simulink model "siso_pitch_break"  (R2026a)
settings: Solver=VariableStepAuto  StopTime=10
undefined symbols (not defined in the file or in its folder): P
libraries: slpidlib x2, dspfdesign x1, simulink x1
settings Model: Creator=devinbellll  LastModifiedBy=devinbellll

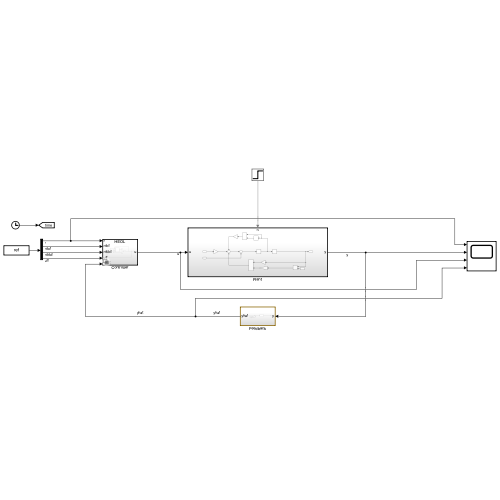
[thumbnail: Simulink's stored preview of the top-level diagram]
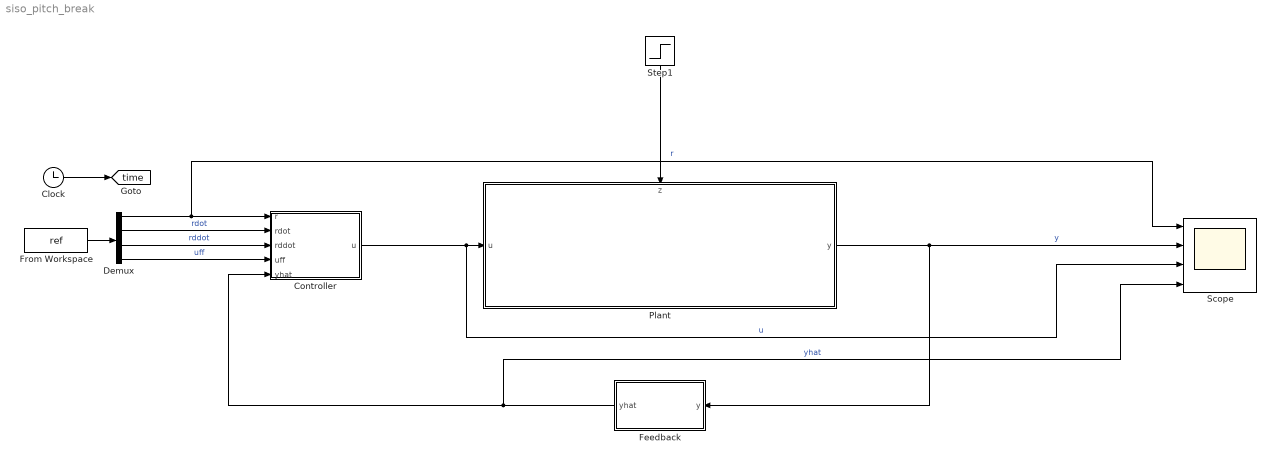
== system siso_pitch_break ==
  Clock : Clock
  Controller : Subsystem  Variant=on  VariantControlMode=label  LabelModeActiveChoice=HEOL
  Demux : Demux
  Feedback : Subsystem
  From Workspace : FromWorkspace  VariableName=ref
  Plant : Subsystem
      settings: PortSchema="{\"entries\":[{\"content\":{\"sides\":[{\"content\":{\"connectorIds\":[\"In1\"]},\"type\":\"ConnectorPlacement.EquallySpacedRectSide\",\"uuid\":\"c97da850-f89b-4091-b1f5-05dae9f68cd3\"},{\"content\":{\"connectorIds\":[\"Out1\"],\"side\":\"RIGHT\"},\"type\":\"ConnectorPlacement.EquallySpacedRectSide\",\"uuid\":\"c303f837-7d2b-4813-8ee2-fdf25e492c4f\"},{\"content\":{\"connectorIds\":[\"In2\"],\"side\":\"TOP\"},\"type\":\"ConnectorPlacement.EquallySpacedRectSide\",\"uuid\":\"7bfe1516-e3c7-473c-aa51-3e09351ce59e\"}]},\"type\":\"ConnectorPlacement.EquallySpacedConnector\",\"uuid\":\"d0f3ac38-9d06-47ac-81ff-254dc0ebc63c\"}],\"packageUris\":[\"http://schema.mathworks.com/mf0/Connector/R2020b\"],\"version\":\"1.0\"}"
  Scope : Scope  NumInputPorts=4
      settings: ActiveDisplayYMinimum=-0.1850564356772344  ActiveDisplayYMaximum=0.35875841753576132
  Step1 : Step  Time=5  FinalValue=10  SampleTime=0
  tag scope: time=global
  wires:
  Plant/1(y) -> Feedback/1(y), Scope/2  "y"
  Clock/1 -> [time]
  Demux/1 -> Controller/1(r), Scope/1  "r"
  Step1/1 -> Plant/2(z)
  Feedback/1(yhat) -> Controller/5(yhat), Scope/4  "yhat"
  From Workspace/1 -> Demux/1
  Demux/2 -> Controller/2(rdot)  "rdot"
  Demux/3 -> Controller/3(rddot)  "rddot"
  Demux/4 -> Controller/4(uff)  "uff"
  Controller/1(u) -> Plant/1(u), Scope/3  "u"

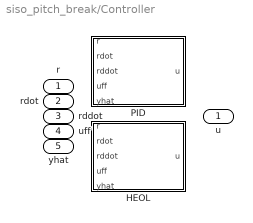
== system siso_pitch_break/Controller ==
  r : Inport
  rdot : Inport  Port=2
  rddot : Inport  Port=3
  uff : Inport  Port=4
  yhat : Inport  Port=5
  HEOL : Subsystem  VariantControl=HEOL
  PID : Subsystem  VariantControl=PID
  u : Outport

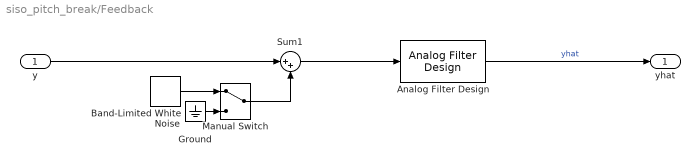
== system siso_pitch_break/Feedback ==
  y : Inport
  Analog Filter Design : dspfdesign/Analog Filter Design  method=Butterworth  filttype=Lowpass  N=2  Wlo=P.wf  Whi=80  Rp=2  Rs=40
  Band-Limited White Noise : simulink/Sources/Band-Limited White Noise  Cov=P.noise_pw  Ts=P.Ts  seed=P.seed
  Ground : Ground
  Manual Switch : ManualSwitch
  Sum1 : Sum  Inputs=|++
  yhat : Outport
  wires:
  y/1 -> Sum1/1
  Manual Switch/1 -> Sum1/2
  Band-Limited White Noise/1 -> Manual Switch/1
  Ground/1 -> Manual Switch/2
  Analog Filter Design/1 -> yhat/1  "yhat"
  Sum1/1 -> Analog Filter Design/1

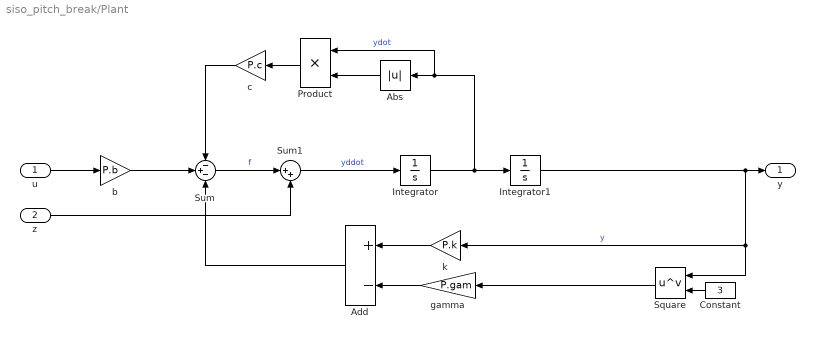
== system siso_pitch_break/Plant ==
  u : Inport
  z : Inport  Port=2
  Abs : Abs  SaturateOnIntegerOverflow=off
  Add : Sum  Inputs=+-
  Constant : Constant  Value=3
  Integrator : Integrator
  Integrator1 : Integrator
  Product : Product
  Square : Math  Operator=pow
  Sum : Sum  Inputs=-+-
  Sum1 : Sum  Inputs=|++
  b : Gain  Gain=P.b
  c : Gain  Gain=P.c
  gamma : Gain  Gain=P.gam
  k : Gain  Gain=P.k
  y : Outport
  wires:
  u/1 -> b/1
  b/1 -> Sum/2
  Abs/1 -> Product/2
  Sum/1 -> Sum1/1  "f"
  Integrator/1 -> Product/1, Abs/1, Integrator1/1  "ydot"
  Integrator1/1 -> Square/1, k/1, y/1  "y"
  Product/1 -> c/1
  c/1 -> Sum/1
  Add/1 -> Sum/3
  gamma/1 -> Add/2
  Square/1 -> gamma/1
  Constant/1 -> Square/2
  k/1 -> Add/1
  Sum1/1 -> Integrator/1  "yddot"
  z/1 -> Sum1/2

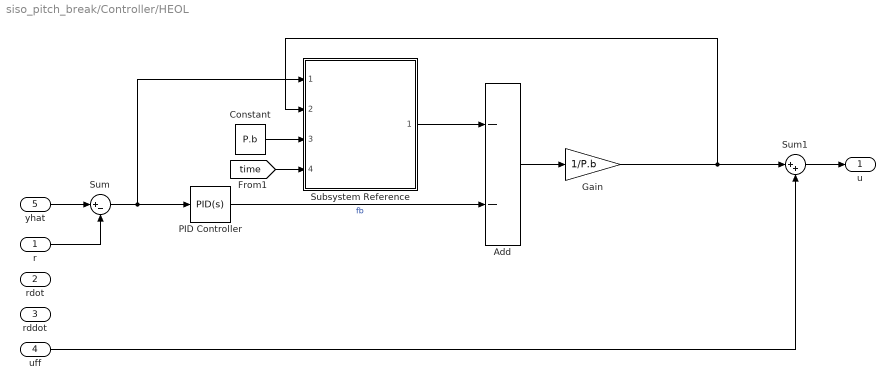
== system siso_pitch_break/Controller/HEOL ==
  r : Inport
  rdot : Inport  Port=2
  rddot : Inport  Port=3
  uff : Inport  Port=4
  yhat : Inport  Port=5
  Add : Sum  Inputs=--
  Constant : Constant  Value=P.b
  Gain : Gain  Gain=1/P.b
  PID Controller : slpidlib/PID Controller  Controller=PID  Form=Parallel  TimeDomain=Continuous-time  UseExternalTs=off  SampleTime=-1  IntegratorMethod=Forward Euler  FilterMethod=Forward Euler  ControllerParametersSource=internal  P=P.Kp  I=P.Ki  UseKiTs=off  D=P.Kd  UseExternalDerivativeSource=off  N=P.N  UseFilter=on  TunerSelectOption=Transfer Function Based (PID Tuner App)  InitialConditionSource=internal  InitialConditionForIntegrator=0  InitialConditionForFilter=0  DifferentiatorICPrevScaledInput=0  ExternalReset=none  TrackingMode=off  Kt=1  LimitOutput=off  SatLimitsSource=internal  UpperSaturationLimit=inf  LowerSaturationLimit=-inf  LinearizeAsGain=on  AntiWindupMode=none  Kb=1  LimitIntegrator=off  UpperIntegratorSaturationLimit=inf  LowerIntegratorSaturationLimit=-inf  POutMin=[]  POutMax=[]  IOutMin=[]  IOutMax=[]  DOutMin=[]  DOutMax=[]  NOutMin=[]  NOutMax=[]  SumOutMin=[]  SumOutMax=[]  SaturationOutMin=[]  SaturationOutMax=[]  PParamMin=[]  PParamMax=[]  IParamMin=[]  IParamMax=[]  DParamMin=[]  DParamMax=[]  NParamMin=[]  NParamMax=[]  KbParamMin=[]  KbParamMax=[]  KtParamMin=[]  KtParamMax=[]  KbOutMin=[]  KbOutMax=[]  KtOutMin=[]  KtOutMax=[]  IntegratorOutMin=[]  IntegratorOutMax=[]  FilterOutMin=[]  FilterOutMax=[]  SumI1OutMin=[]  SumI1OutMax=[]  SumI2OutMin=[]  SumI2OutMax=[]  SumI3OutMin=[]  SumI3OutMax=[]  SumI4OutMin=[]  SumI4OutMax=[]  SumDOutMin=[]  SumDOutMax=[]  DifferentiatorOutMin=[]  DifferentiatorOutMax=[]  FilterDiffOutCoefMin=[]  FilterDiffOutCoefMax=[]  ReciprocalOutMin=[]  ReciprocalOutMax=[]  SumDenOutMin=[]  SumDenOutMax=[]  SumNumOutMin=[]  SumNumOutMax=[]  DivideOutMin=[]  DivideOutMax=[]  UdiffTsProdOutMin=[]  UdiffTsProdOutMax=[]  NTsProdOutMin=[]  NTsProdOutMax=[]  UintegralTsProdOutMin=[]  UintegralTsProdOutMax=[]  UngainTsProdOutMin=[]  UngainTsProdOutMax=[]  ClampingZeroOutDataTypeStr=Inherit: Inherit via back propagation  ClampingZeroOutMin=[]  ClampingZeroOutMax=[]  FilterDenConstantOutDataTypeStr=Inherit: Inherit via back propagation  FilterDenConstantOutMin=[]  FilterDenConstantOutMax=[]  PCopyOutDataTypeStr=Inherit: Inherit via back propagation  PCopyOutMin=[]  PCopyOutMax=[]  NCopyOutDataTypeStr=Inherit: Inherit via back propagation  NCopyOutMin=[]  NCopyOutMax=[]  IntegratorContinuousStateAttributes=''  IntegratorStateMustResolveToSignalObject=off  IntegratorRTWStateStorageClass=Auto  FilterContinuousStateAttributes=''  FilterStateMustResolveToSignalObject=off  FilterRTWStateStorageClass=Auto  ParallelPVariant=InternalParameters  IdealPVariant=Disabled  IVariant=InternalParameters  DVariant=InternalParameters  IntegratorVariant=Continuous  SatVariant=Disabled  AWVariant=Passthrough  PCopyVariant=Disabled  TRVariant=Disabled  FdbkBlocksVariant=Forward  IdealPFdbkVariant=Disabled  SatFdbkVariant=Disabled  DerivativeFilterVariant=ContFilter  NVariant=InternalParameters  NCopyVariant=Disabled  FilterICVariant=InternalICsFilter  IntegratorICVariant=InternalICs  ExternalResetVariant=Disabled  TRSumVariant=Passthrough  SumFdbkVariant=Disabled  SumVariant=Sum_PID  TsampFilterVariant=InternalTs  TsampNgainVariant=Passthrough  TsampIntegralVariant=Disabled_SignalSpec  ExternalSaturationOutDataTypeStr=Inherit: Same as second input  DerivativeSourceVariant=ErrorSignal  PreIntVariant=InternalPreInt
  Subsystem Reference : Subsystem  ReferencedSubsystem=mfc_F_est_cont
  Sum : Sum  Inputs=|+-
  Sum1 : Sum  Inputs=|++
  u : Outport
  wires:
  uff/1 -> Sum1/2
  Sum1/1 -> u/1
  PID Controller/1 -> Add/2  "fb"
  r/1 -> Sum/2
  Sum/1 -> Subsystem Reference/1, PID Controller/1
  [time] -> Subsystem Reference/4
  yhat/1 -> Sum/1
  Constant/1 -> Subsystem Reference/3
  Gain/1 -> Subsystem Reference/2, Sum1/1
  Subsystem Reference/1 -> Add/1
  Add/1 -> Gain/1

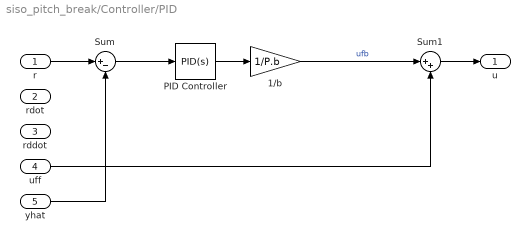
== system siso_pitch_break/Controller/PID ==
  r : Inport
  rdot : Inport  Port=2
  rddot : Inport  Port=3
  uff : Inport  Port=4
  yhat : Inport  Port=5
  1/b : Gain  Gain=1/P.b
  PID Controller : slpidlib/PID Controller  Controller=PID  Form=Parallel  TimeDomain=Continuous-time  UseExternalTs=off  SampleTime=-1  IntegratorMethod=Forward Euler  FilterMethod=Forward Euler  ControllerParametersSource=internal  P=P.Kp  I=P.Ki  UseKiTs=off  D=P.Kd  UseExternalDerivativeSource=off  N=P.N  UseFilter=on  TunerSelectOption=Transfer Function Based (PID Tuner App)  InitialConditionSource=internal  InitialConditionForIntegrator=0  InitialConditionForFilter=0  DifferentiatorICPrevScaledInput=0  ExternalReset=none  TrackingMode=off  Kt=1  LimitOutput=off  SatLimitsSource=internal  UpperSaturationLimit=inf  LowerSaturationLimit=-inf  LinearizeAsGain=on  AntiWindupMode=none  Kb=1  LimitIntegrator=off  UpperIntegratorSaturationLimit=inf  LowerIntegratorSaturationLimit=-inf  POutMin=[]  POutMax=[]  IOutMin=[]  IOutMax=[]  DOutMin=[]  DOutMax=[]  NOutMin=[]  NOutMax=[]  SumOutMin=[]  SumOutMax=[]  SaturationOutMin=[]  SaturationOutMax=[]  PParamMin=[]  PParamMax=[]  IParamMin=[]  IParamMax=[]  DParamMin=[]  DParamMax=[]  NParamMin=[]  NParamMax=[]  KbParamMin=[]  KbParamMax=[]  KtParamMin=[]  KtParamMax=[]  KbOutMin=[]  KbOutMax=[]  KtOutMin=[]  KtOutMax=[]  IntegratorOutMin=[]  IntegratorOutMax=[]  FilterOutMin=[]  FilterOutMax=[]  SumI1OutMin=[]  SumI1OutMax=[]  SumI2OutMin=[]  SumI2OutMax=[]  SumI3OutMin=[]  SumI3OutMax=[]  SumI4OutMin=[]  SumI4OutMax=[]  SumDOutMin=[]  SumDOutMax=[]  DifferentiatorOutMin=[]  DifferentiatorOutMax=[]  FilterDiffOutCoefMin=[]  FilterDiffOutCoefMax=[]  ReciprocalOutMin=[]  ReciprocalOutMax=[]  SumDenOutMin=[]  SumDenOutMax=[]  SumNumOutMin=[]  SumNumOutMax=[]  DivideOutMin=[]  DivideOutMax=[]  UdiffTsProdOutMin=[]  UdiffTsProdOutMax=[]  NTsProdOutMin=[]  NTsProdOutMax=[]  UintegralTsProdOutMin=[]  UintegralTsProdOutMax=[]  UngainTsProdOutMin=[]  UngainTsProdOutMax=[]  ClampingZeroOutDataTypeStr=Inherit: Inherit via back propagation  ClampingZeroOutMin=[]  ClampingZeroOutMax=[]  FilterDenConstantOutDataTypeStr=Inherit: Inherit via back propagation  FilterDenConstantOutMin=[]  FilterDenConstantOutMax=[]  PCopyOutDataTypeStr=Inherit: Inherit via back propagation  PCopyOutMin=[]  PCopyOutMax=[]  NCopyOutDataTypeStr=Inherit: Inherit via back propagation  NCopyOutMin=[]  NCopyOutMax=[]  IntegratorContinuousStateAttributes=''  IntegratorStateMustResolveToSignalObject=off  IntegratorRTWStateStorageClass=Auto  FilterContinuousStateAttributes=''  FilterStateMustResolveToSignalObject=off  FilterRTWStateStorageClass=Auto  ParallelPVariant=InternalParameters  IdealPVariant=Disabled  IVariant=InternalParameters  DVariant=InternalParameters  IntegratorVariant=Continuous  SatVariant=Disabled  AWVariant=Passthrough  PCopyVariant=Disabled  TRVariant=Disabled  FdbkBlocksVariant=Forward  IdealPFdbkVariant=Disabled  SatFdbkVariant=Disabled  DerivativeFilterVariant=ContFilter  NVariant=InternalParameters  NCopyVariant=Disabled  FilterICVariant=InternalICsFilter  IntegratorICVariant=InternalICs  ExternalResetVariant=Disabled  TRSumVariant=Passthrough  SumFdbkVariant=Disabled  SumVariant=Sum_PID  TsampFilterVariant=InternalTs  TsampNgainVariant=Passthrough  TsampIntegralVariant=Disabled_SignalSpec  ExternalSaturationOutDataTypeStr=Inherit: Same as second input  DerivativeSourceVariant=ErrorSignal  PreIntVariant=InternalPreInt
  Sum : Sum  Inputs=|+-
  Sum1 : Sum  Inputs=|++
  u : Outport
  wires:
  Sum/1 -> PID Controller/1
  yhat/1 -> Sum/2
  1/b/1 -> Sum1/1  "ufb"
  r/1 -> Sum/1
  PID Controller/1 -> 1/b/1
  Sum1/1 -> u/1
  uff/1 -> Sum1/2
